simulink model "hip_controller_2026_03_03"  (R2024b)
settings: Solver=FixedStepAuto  StartTime=0.0  StopTime=simDuration  FixedStep=0.01  RelTol=1e-3  EnableMultiTasking=on
InitFcn:
  | breakp=[-1, -0.8, -0.6, -0.4, -0.2, -0.1, 0, 0.1, 0.2, 0.4, 0.6, 0.8, 1];
  | splinenew =[-1, -0.8, -0.6, -0.4, -0.2, -0.1, 0, 0, 0.005, 0.01, 0.015,0.02,0.025];
undefined symbols (not defined in the file or in its folder): Discrete, K, qbreak, Time
libraries: simulink x121, arduinolib x41, dspswit3 x21, ctrlSharedLib x2, dspfdesign x2, slpidlib x2
(part 4 of 7)

== system hip_controller_2026_03_03/Subsystem6/Right Motor Velocity/Subsystem ==
  Motor command : Inport
  SWITCH : Inport  Port=2
  CAN Pack1 : Subsystem
  CAN Transmit1 : arduinolib/CAN Transmit  Priority=1  inputDataType=Raw data  BlockingMode_=on  BlockTimeout_=1  outputStatus=off  identifierType=Standard (11-bit identifier)  messageId=3  msgLength=8  remoteFrame=off
      settings: SourceProductName=Common
  Constant7 : Constant  Value=0  OutDataTypeStr=single  SampleTime=0.01
  DISABLE1 : Constant  Value=269.7/18  OutDataTypeStr=single
  Data Type Conversion3 : DataTypeConversion  OutDataTypeStr=single  SaturateOnIntegerOverflow=off  RndMeth=Floor
  Demux1 : Demux  Outputs=5
  ENABLE1 : Constant  Value=14.975  OutDataTypeStr=single
  IsNaN : RelationalOperator  Operator=isNaN  OutDataTypeStr=boolean  RndMeth=Simplest  InputSameDT=off
  N-Sample Switch4 : dspswit3/N-Sample Switch  N=15  reset=on  TriggerType=Either edge  Ts=0.01
  Rate Transition : RateTransition  OutPortSampleTime=0.01
  Subsystem2 : Subsystem
  Switch : Switch  Criteria=u2 > Threshold  SaturateOnIntegerOverflow=off  InputSameDT=off
  Switch3 : Switch  Criteria=u2 > Threshold  SaturateOnIntegerOverflow=off  InputSameDT=off
  wires:
  Demux1/4 -> CAN Pack1/4(Kd)
  Data Type Conversion3/1 -> Subsystem2/2(Velocity)
  Switch3/1 -> Subsystem2/1(Enable)
  Demux1/1 -> CAN Pack1/1(Position)
  Motor command/1 -> Data Type Conversion3/1, IsNaN/1
  Demux1/5 -> CAN Pack1/5(Torque)
  ENABLE1/1 -> Switch3/1
  Demux1/2 -> CAN Pack1/2(Velocity)
  Rate Transition/1 -> N-Sample Switch4/3
  IsNaN/1 -> Switch/2
  DISABLE1/1 -> Switch3/3
  Subsystem2/1(Enter_motor_mode) -> N-Sample Switch4/1
  Demux1/3 -> CAN Pack1/3(Kp)
  N-Sample Switch4/1 -> Demux1/1
  Switch/1 -> Rate Transition/1, Switch3/2
  CAN Pack1/1(CAN Data) -> CAN Transmit1/1
  Subsystem2/2(Velocity_value) -> N-Sample Switch4/2
  Constant7/1 -> Switch/1
  SWITCH/1 -> Switch/3

== system hip_controller_2026_03_03/Initialize Function/Config_L /X=Z, Y=Y, Z=X/Enabled Subsystem ==
  Enable : EnablePort
  Compare To Constant1 : simulink/Logic and Bit Operations/Compare To Constant  relop===  const=0  OutDataTypeStr=boolean
  Constant2 : Constant  Value=0x06
  I2C Write6 : arduinolib/I2C Write  I2CModule=0  Mode=Master  SlaveAddress=0x28  SlaveByteOrder=BigEndian  Direction=Transmitter  RegisterAddressMode=on  RegisterAddress=0x41  SlaveDataType=uint8  DataLength=1  NoAck=off  RepeatedStart=off  OutputStatus=on  blockPlatform=ARDUINO
      settings: SourceProductName=Common
  Status : Outport
  wires:
  Constant2/1 -> I2C Write6/1
  I2C Write6/1 -> Compare To Constant1/1  "0: success"
  Compare To Constant1/1 -> Status/1

== system hip_controller_2026_03_03/Initialize Function/Config_L /Z = -Z/Write ==
  Enable : EnablePort
  Compare To Constant1 : simulink/Logic and Bit Operations/Compare To Constant  relop===  const=0  OutDataTypeStr=boolean
  Constant2 : Constant  Value=0x01
  I2C Write7 : arduinolib/I2C Write  I2CModule=0  Mode=Master  SlaveAddress=0x28  SlaveByteOrder=BigEndian  Direction=Transmitter  RegisterAddressMode=on  RegisterAddress=0x42  SlaveDataType=uint8  DataLength=1  NoAck=off  RepeatedStart=off  OutputStatus=on  blockPlatform=ARDUINO
      settings: SourceProductName=Common
  Status : Outport
  wires:
  Constant2/1 -> I2C Write7/1
  I2C Write7/1 -> Compare To Constant1/1  "0: success"
  Compare To Constant1/1 -> Status/1

== system hip_controller_2026_03_03/Initialize Function/Config_R/X=Z, Y=Y, Z=X/Enabled Subsystem ==
  Enable : EnablePort
  Compare To Constant1 : simulink/Logic and Bit Operations/Compare To Constant  relop===  const=0  OutDataTypeStr=boolean
  Constant2 : Constant  Value=0x06
  I2C Write6 : arduinolib/I2C Write  I2CModule=0  Mode=Master  SlaveAddress=0x29  SlaveByteOrder=BigEndian  Direction=Transmitter  RegisterAddressMode=on  RegisterAddress=0x41  SlaveDataType=uint8  DataLength=1  NoAck=off  RepeatedStart=off  OutputStatus=on  blockPlatform=ARDUINO
      settings: SourceProductName=Common
  Status : Outport
  wires:
  Constant2/1 -> I2C Write6/1
  I2C Write6/1 -> Compare To Constant1/1  "0: success"
  Compare To Constant1/1 -> Status/1

== system hip_controller_2026_03_03/Initialize Function/Config_R/Z = -Z/Write ==
  Enable : EnablePort
  Compare To Constant1 : simulink/Logic and Bit Operations/Compare To Constant  relop===  const=0  OutDataTypeStr=boolean
  Constant2 : Constant  Value=0x01
  I2C Write7 : arduinolib/I2C Write  I2CModule=0  Mode=Master  SlaveAddress=0x29  SlaveByteOrder=BigEndian  Direction=Transmitter  RegisterAddressMode=on  RegisterAddress=0x42  SlaveDataType=uint8  DataLength=1  NoAck=off  RepeatedStart=off  OutputStatus=on  blockPlatform=ARDUINO
      settings: SourceProductName=Common
  Status : Outport
  wires:
  Constant2/1 -> I2C Write7/1
  I2C Write7/1 -> Compare To Constant1/1  "0: success"
  Compare To Constant1/1 -> Status/1

== system hip_controller_2026_03_03/LEFT LEG1/Pos and Vel normalized/Subsystem4/If Action Subsystem ==
  Clock : Inport
  angle : Inport  Port=2
  Action Port : ActionPort
  Compare To Constant1 : simulink/Logic and Bit Operations/Compare To Constant  relop=>=  const=0.3  OutDataTypeStr=boolean
  Enabled Subsystem : Subsystem  TreatAsAtomicUnit=on
  Memory : Memory  InheritSampleTime=on
  Subtract : Sum  Inputs=+-
  Zero-Order Hold : ZeroOrderHold  SampleTime=-1
  Angle_max : Outport
  wires:
  Subtract/1 -> Compare To Constant1/1  "diff"
  Compare To Constant1/1 -> Enabled Subsystem/Enable  "enable"
  Enabled Subsystem/1(angle_out) -> Angle_max/1  "angle_out"
  angle/1 -> Enabled Subsystem/1(angle_in)
  Clock/1 -> Zero-Order Hold/1  "clock"
  Zero-Order Hold/1 -> Subtract/1, Memory/1  "clock_ZOH"
  Memory/1 -> Subtract/2  "clock_memory"

== system hip_controller_2026_03_03/LEFT LEG1/Pos and Vel normalized/Subsystem5/If Action Subsystem ==
  Angle : Inport
  Clock : Inport  Port=2
  Action Port : ActionPort
  Compare To Constant1 : simulink/Logic and Bit Operations/Compare To Constant  relop=>=  const=0.3  OutDataTypeStr=boolean
  Enabled Subsystem : Subsystem  TreatAsAtomicUnit=on
  Memory : Memory  InheritSampleTime=on
  Subtract : Sum  Inputs=+-
  Zero-Order Hold : ZeroOrderHold  SampleTime=-1
  Angle_min : Outport
  wires:
  Memory/1 -> Subtract/2  "clock_memory"
  Zero-Order Hold/1 -> Subtract/1, Memory/1  "clock_ZOH"
  Enabled Subsystem/1(angle_out) -> Angle_min/1  "angle_out"
  Compare To Constant1/1 -> Enabled Subsystem/Enable  "enable"
  Clock/1 -> Zero-Order Hold/1  "clock"
  Subtract/1 -> Compare To Constant1/1  "diff"
  Angle/1 -> Enabled Subsystem/1(angle_in)

== system hip_controller_2026_03_03/LEFT LEG1/Pos and Vel normalized/Subsystem6/If Action Subsystem ==
  Velocity : Inport
  Clock : Inport  Port=2
  Action Port : ActionPort
  Compare To Constant1 : simulink/Logic and Bit Operations/Compare To Constant  relop=>=  const=0.3  OutDataTypeStr=boolean
  Enabled Subsystem : Subsystem  TreatAsAtomicUnit=on
  Memory : Memory  InheritSampleTime=on
  Subtract : Sum  Inputs=+-
  Zero-Order Hold : ZeroOrderHold  SampleTime=-1
  Vel_min : Outport
  wires:
  Enabled Subsystem/1(vel_out) -> Vel_min/1  "angle_out"
  Memory/1 -> Subtract/2  "clock_memory"
  Velocity/1 -> Enabled Subsystem/1(vel_in)
  Zero-Order Hold/1 -> Subtract/1, Memory/1  "clock_ZOH"
  Clock/1 -> Zero-Order Hold/1  "clock"
  Subtract/1 -> Compare To Constant1/1  "diff"
  Compare To Constant1/1 -> Enabled Subsystem/Enable  "enable"

== system hip_controller_2026_03_03/LEFT LEG1/Pos and Vel normalized/Subsystem7/If Action Subsystem ==
  Velocity : Inport
  Clock : Inport  Port=2
  Action Port : ActionPort
  Compare To Constant1 : simulink/Logic and Bit Operations/Compare To Constant  relop=>=  const=0.3  OutDataTypeStr=boolean
  Enabled Subsystem : Subsystem  TreatAsAtomicUnit=on
  Memory : Memory  InheritSampleTime=on
  Subtract : Sum  Inputs=+-
  Zero-Order Hold : ZeroOrderHold  SampleTime=-1
  Vel_max : Outport
  wires:
  Memory/1 -> Subtract/2  "clock_memory"
  Compare To Constant1/1 -> Enabled Subsystem/Enable  "enable"
  Clock/1 -> Zero-Order Hold/1  "clock"
  Zero-Order Hold/1 -> Subtract/1, Memory/1  "clock_ZOH"
  Enabled Subsystem/1(vel_out) -> Vel_max/1  "angle_out"
  Subtract/1 -> Compare To Constant1/1  "diff"
  Velocity/1 -> Enabled Subsystem/1(vel_in)

== system hip_controller_2026_03_03/RIGHT_LEG1/Pos and Vel normalized/Subsystem4/If Action Subsystem ==
  Clock : Inport
  angle : Inport  Port=2
  Action Port : ActionPort
  Compare To Constant1 : simulink/Logic and Bit Operations/Compare To Constant  relop=>=  const=0.3  OutDataTypeStr=boolean
  Enabled Subsystem : Subsystem  TreatAsAtomicUnit=on
  Memory : Memory  InheritSampleTime=on
  Subtract : Sum  Inputs=+-
  Zero-Order Hold : ZeroOrderHold  SampleTime=-1
  Angle_max : Outport
  wires:
  Subtract/1 -> Compare To Constant1/1  "diff"
  Compare To Constant1/1 -> Enabled Subsystem/Enable  "enable"
  Enabled Subsystem/1(angle_out) -> Angle_max/1  "angle_out"
  angle/1 -> Enabled Subsystem/1(angle_in)
  Clock/1 -> Zero-Order Hold/1  "clock"
  Zero-Order Hold/1 -> Subtract/1, Memory/1  "clock_ZOH"
  Memory/1 -> Subtract/2  "clock_memory"

== system hip_controller_2026_03_03/RIGHT_LEG1/Pos and Vel normalized/Subsystem5/If Action Subsystem ==
  Angle : Inport
  Clock : Inport  Port=2
  Action Port : ActionPort
  Compare To Constant1 : simulink/Logic and Bit Operations/Compare To Constant  relop=>=  const=0.3  OutDataTypeStr=boolean
  Enabled Subsystem : Subsystem  TreatAsAtomicUnit=on
  Memory : Memory  InheritSampleTime=on
  Subtract : Sum  Inputs=+-
  Zero-Order Hold : ZeroOrderHold  SampleTime=-1
  Angle_min : Outport
  wires:
  Memory/1 -> Subtract/2  "clock_memory"
  Zero-Order Hold/1 -> Subtract/1, Memory/1  "clock_ZOH"
  Enabled Subsystem/1(angle_out) -> Angle_min/1  "angle_out"
  Compare To Constant1/1 -> Enabled Subsystem/Enable  "enable"
  Clock/1 -> Zero-Order Hold/1  "clock"
  Subtract/1 -> Compare To Constant1/1  "diff"
  Angle/1 -> Enabled Subsystem/1(angle_in)

== system hip_controller_2026_03_03/RIGHT_LEG1/Pos and Vel normalized/Subsystem6/If Action Subsystem ==
  Velocity : Inport
  Clock : Inport  Port=2
  Action Port : ActionPort
  Compare To Constant1 : simulink/Logic and Bit Operations/Compare To Constant  relop=>=  const=0.3  OutDataTypeStr=boolean
  Enabled Subsystem : Subsystem  TreatAsAtomicUnit=on
  Memory : Memory  InheritSampleTime=on
  Subtract : Sum  Inputs=+-
  Zero-Order Hold : ZeroOrderHold  SampleTime=-1
  Vel_min : Outport
  wires:
  Enabled Subsystem/1(vel_out) -> Vel_min/1  "angle_out"
  Memory/1 -> Subtract/2  "clock_memory"
  Velocity/1 -> Enabled Subsystem/1(vel_in)
  Zero-Order Hold/1 -> Subtract/1, Memory/1  "clock_ZOH"
  Clock/1 -> Zero-Order Hold/1  "clock"
  Subtract/1 -> Compare To Constant1/1  "diff"
  Compare To Constant1/1 -> Enabled Subsystem/Enable  "enable"

== system hip_controller_2026_03_03/RIGHT_LEG1/Pos and Vel normalized/Subsystem7/If Action Subsystem ==
  Velocity : Inport
  Clock : Inport  Port=2
  Action Port : ActionPort
  Compare To Constant1 : simulink/Logic and Bit Operations/Compare To Constant  relop=>=  const=0.3  OutDataTypeStr=boolean
  Enabled Subsystem : Subsystem  TreatAsAtomicUnit=on
  Memory : Memory  InheritSampleTime=on
  Subtract : Sum  Inputs=+-
  Zero-Order Hold : ZeroOrderHold  SampleTime=-1
  Vel_max : Outport
  wires:
  Memory/1 -> Subtract/2  "clock_memory"
  Compare To Constant1/1 -> Enabled Subsystem/Enable  "enable"
  Clock/1 -> Zero-Order Hold/1  "clock"
  Zero-Order Hold/1 -> Subtract/1, Memory/1  "clock_ZOH"
  Enabled Subsystem/1(vel_out) -> Vel_max/1  "angle_out"
  Subtract/1 -> Compare To Constant1/1  "diff"
  Velocity/1 -> Enabled Subsystem/1(vel_in)

== system hip_controller_2026_03_03/Subsystem3/Left Motor Velocity/Motor Actual Position Receive/CHINESE CORRECTION ==
  position : Inport
  Enable : EnablePort  StatesWhenEnabling=reset
  Abs : Abs  SaturateOnIntegerOverflow=off
  Constant2 : Constant
  Constant3 : Constant  Value=0
  Memory : Memory
  Subsystem : Subsystem
  Sum : Sum  Inputs=|+-
  Sum1 : Sum  Inputs=+-
  Switch1 : Switch  Criteria=u2 > Threshold  Threshold=20  SaturateOnIntegerOverflow=off  InputSameDT=off
  Out1 : Outport
  wires:
  Constant2/1 -> Switch1/1
  position/1 -> Sum1/1, Sum/1, Memory/1
  Sum/1 -> Abs/1, Subsystem/1(In1)
  Sum1/1 -> Out1/1
  Abs/1 -> Switch1/2
  Constant3/1 -> Switch1/3
  Switch1/1 -> Subsystem/Enable
  Memory/1 -> Sum/2
  Subsystem/1(Out1) -> Sum1/2

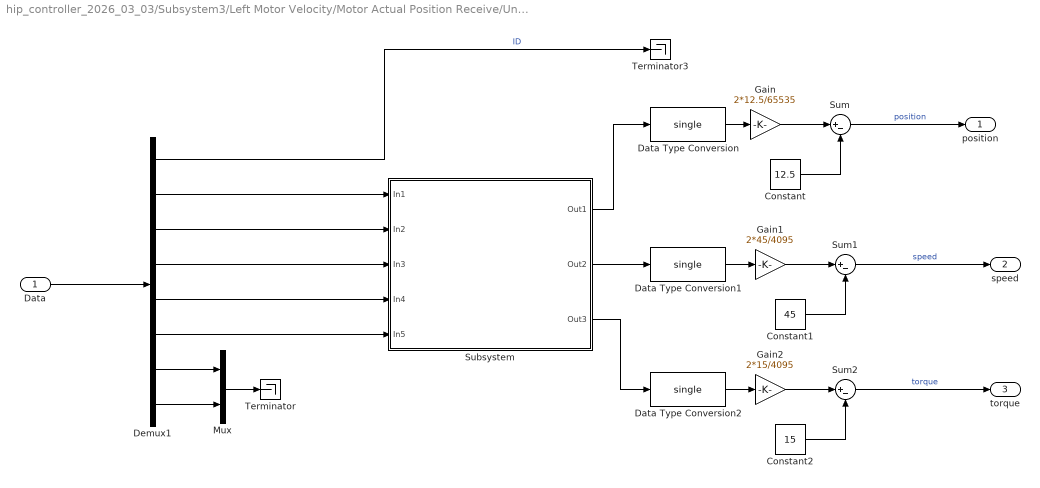
== system hip_controller_2026_03_03/Subsystem3/Left Motor Velocity/Motor Actual Position Receive/Unpack2 ==
  Data : Inport
  Constant : Constant  Value=12.5
  Constant1 : Constant  Value=45
  Constant2 : Constant  Value=15
  Data Type Conversion : DataTypeConversion  OutDataTypeStr=single  SaturateOnIntegerOverflow=off  RndMeth=Floor
  Data Type Conversion1 : DataTypeConversion  OutDataTypeStr=single  SaturateOnIntegerOverflow=off  RndMeth=Floor
  Data Type Conversion2 : DataTypeConversion  OutDataTypeStr=single  SaturateOnIntegerOverflow=off  RndMeth=Floor
  Demux1 : Demux  Outputs=8
  Gain : Gain  Gain=2*12.5/65535  RndMeth=Round
  Gain1 : Gain  Gain=2*45/4095  RndMeth=Round
  Gain2 : Gain  Gain=2*15/4095  RndMeth=Round
  Mux : Mux  Inputs=2
  Subsystem : Subsystem
  Sum : Sum  Inputs=|+-
  Sum1 : Sum  Inputs=|+-
  Sum2 : Sum  Inputs=|+-
  Terminator : Terminator
  Terminator3 : Terminator
  position : Outport
  speed : Outport  Port=2
  torque : Outport  Port=3
  wires:
  Demux1/1 -> Terminator3/1  "ID"
  Demux1/7 -> Mux/1
  Demux1/8 -> Mux/2
  Demux1/2 -> Subsystem/1(In1)
  Demux1/3 -> Subsystem/2(In2)
  Demux1/4 -> Subsystem/3(In3)
  Demux1/5 -> Subsystem/4(In4)
  Demux1/6 -> Subsystem/5(In5)
  Subsystem/1(Out1) -> Data Type Conversion/1
  Gain/1 -> Sum/1
  Constant/1 -> Sum/2
  Data Type Conversion/1 -> Gain/1
  Gain1/1 -> Sum1/1
  Data Type Conversion1/1 -> Gain1/1
  Constant1/1 -> Sum1/2
  Gain2/1 -> Sum2/1
  Data Type Conversion2/1 -> Gain2/1
  Constant2/1 -> Sum2/2
  Subsystem/2(Out2) -> Data Type Conversion1/1
  Subsystem/3(Out3) -> Data Type Conversion2/1
  Sum2/1 -> torque/1  "torque"
  Mux/1 -> Terminator/1
  Data/1 -> Demux1/1
  Sum/1 -> position/1  "position"
  Sum1/1 -> speed/1  "speed"

== system hip_controller_2026_03_03/Subsystem3/Left Motor Velocity/Subsystem/CAN Pack1 ==
  Position : Inport
  Velocity : Inport  Port=2
  Kp : Inport  Port=3
  Kd : Inport  Port=4
  Torque : Inport  Port=5
  Constant3 : Constant  Value=-12.5  OutDataTypeStr=single
  Constant4 : Constant  Value=-45  OutDataTypeStr=single
  Constant5 : Constant  Value=-15  OutDataTypeStr=single
  Gain : Gain  Gain=65535/(2*12.5)  OutDataTypeStr=uint16  RndMeth=Round
  Gain3 : Gain  Gain=4095/(2*45)  OutDataTypeStr=fixdt(0,12,0)  RndMeth=Round
  Gain4 : Gain  Gain=4095/500  OutDataTypeStr=fixdt(0,12,0)  RndMeth=Round
  Gain5 : Gain  Gain=4095/5  OutDataTypeStr=fixdt(0,12,0)  RndMeth=Round
  Gain6 : Gain  Gain=4095/(2*15)  OutDataTypeStr=fixdt(0,12,0)  RndMeth=Round
  Subsystem : Subsystem
  Sum3 : Sum  Inputs=|+-
  Sum4 : Sum  Inputs=|+-
  Sum5 : Sum  Inputs=|+-
  Vector Concatenate : Concatenate  NumInputs=8
  CAN Data : Outport
  wires:
  Velocity/1 -> Sum4/1
  Kp/1 -> Gain4/1
  Kd/1 -> Gain5/1
  Vector Concatenate/1 -> CAN Data/1
  Constant3/1 -> Sum3/2
  Sum3/1 -> Gain/1  "position"
  Position/1 -> Sum3/1
  Constant4/1 -> Sum4/2
  Constant5/1 -> Sum5/2
  Sum5/1 -> Gain6/1  "torque"
  Torque/1 -> Sum5/1
  Sum4/1 -> Gain3/1  "speed"
  Gain/1 -> Subsystem/1(p_int)
  Gain3/1 -> Subsystem/2(v_int)
  Gain4/1 -> Subsystem/3(kp_int)
  Gain5/1 -> Subsystem/4(kd_int)
  Gain6/1 -> Subsystem/5(t_int)
  Subsystem/1(Out2) -> Vector Concatenate/1
  Subsystem/2(Out1) -> Vector Concatenate/2
  Subsystem/4(Out4) -> Vector Concatenate/4
  Subsystem/5(Out5) -> Vector Concatenate/5
  Subsystem/6(Out6) -> Vector Concatenate/6
  Subsystem/7(Out7) -> Vector Concatenate/7
  Subsystem/3(Out3) -> Vector Concatenate/3
  Subsystem/8(Out8) -> Vector Concatenate/8

== system hip_controller_2026_03_03/Subsystem3/Left Motor Velocity/Subsystem/Subsystem2 ==
  Enable : Inport
  Velocity : Inport  Port=2
  Mux1 : Mux  Inputs=5
  Subsystem : Subsystem
  Subsystem2 : Subsystem
  Enter_motor_mode : Outport
  Velocity_value : Outport  Port=2
  wires:
  Subsystem2/3(Out3) -> Mux1/3
  Subsystem2/2(Out2) -> Mux1/2
  Subsystem2/4(Out4) -> Mux1/4
  Subsystem2/1(Out1) -> Mux1/1
  Subsystem/1(Out1) -> Velocity_value/1
  Mux1/1 -> Enter_motor_mode/1
  Enable/1 -> Mux1/5
  Velocity/1 -> Subsystem/1(In1)

== system hip_controller_2026_03_03/Subsystem3/Right Motor Velocity/Motor Actual Position Receive/CHINESE CORRECTION ==
  position : Inport
  Enable : EnablePort  StatesWhenEnabling=reset
  Abs : Abs  SaturateOnIntegerOverflow=off
  Constant2 : Constant
  Constant3 : Constant  Value=0
  Memory : Memory
  Subsystem : Subsystem
  Sum : Sum  Inputs=|+-
  Sum1 : Sum  Inputs=+-
  Switch1 : Switch  Criteria=u2 > Threshold  Threshold=20  SaturateOnIntegerOverflow=off  InputSameDT=off
  Out1 : Outport
  wires:
  Constant2/1 -> Switch1/1
  position/1 -> Sum1/1, Sum/1, Memory/1
  Sum/1 -> Abs/1, Subsystem/1(In1)
  Sum1/1 -> Out1/1
  Abs/1 -> Switch1/2
  Constant3/1 -> Switch1/3
  Switch1/1 -> Subsystem/Enable
  Memory/1 -> Sum/2
  Subsystem/1(Out1) -> Sum1/2

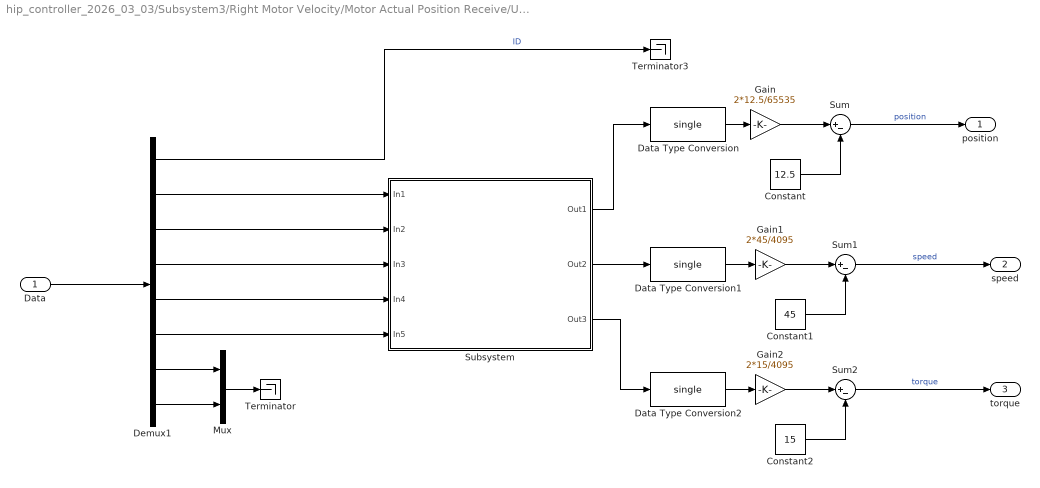
== system hip_controller_2026_03_03/Subsystem3/Right Motor Velocity/Motor Actual Position Receive/Unpack2 ==
  Data : Inport
  Constant : Constant  Value=12.5
  Constant1 : Constant  Value=45
  Constant2 : Constant  Value=15
  Data Type Conversion : DataTypeConversion  OutDataTypeStr=single  SaturateOnIntegerOverflow=off  RndMeth=Floor
  Data Type Conversion1 : DataTypeConversion  OutDataTypeStr=single  SaturateOnIntegerOverflow=off  RndMeth=Floor
  Data Type Conversion2 : DataTypeConversion  OutDataTypeStr=single  SaturateOnIntegerOverflow=off  RndMeth=Floor
  Demux1 : Demux  Outputs=8
  Gain : Gain  Gain=2*12.5/65535  RndMeth=Round
  Gain1 : Gain  Gain=2*45/4095  RndMeth=Round
  Gain2 : Gain  Gain=2*15/4095  RndMeth=Round
  Mux : Mux  Inputs=2
  Subsystem : Subsystem
  Sum : Sum  Inputs=|+-
  Sum1 : Sum  Inputs=|+-
  Sum2 : Sum  Inputs=|+-
  Terminator : Terminator
  Terminator3 : Terminator
  position : Outport
  speed : Outport  Port=2
  torque : Outport  Port=3
  wires:
  Demux1/1 -> Terminator3/1  "ID"
  Demux1/7 -> Mux/1
  Demux1/8 -> Mux/2
  Demux1/2 -> Subsystem/1(In1)
  Demux1/3 -> Subsystem/2(In2)
  Demux1/4 -> Subsystem/3(In3)
  Demux1/5 -> Subsystem/4(In4)
  Demux1/6 -> Subsystem/5(In5)
  Subsystem/1(Out1) -> Data Type Conversion/1
  Gain/1 -> Sum/1
  Constant/1 -> Sum/2
  Data Type Conversion/1 -> Gain/1
  Gain1/1 -> Sum1/1
  Data Type Conversion1/1 -> Gain1/1
  Constant1/1 -> Sum1/2
  Gain2/1 -> Sum2/1
  Data Type Conversion2/1 -> Gain2/1
  Constant2/1 -> Sum2/2
  Subsystem/2(Out2) -> Data Type Conversion1/1
  Subsystem/3(Out3) -> Data Type Conversion2/1
  Sum2/1 -> torque/1  "torque"
  Mux/1 -> Terminator/1
  Data/1 -> Demux1/1
  Sum/1 -> position/1  "position"
  Sum1/1 -> speed/1  "speed"

== system hip_controller_2026_03_03/Subsystem3/Right Motor Velocity/Subsystem/CAN Pack1 ==
  Position : Inport
  Velocity : Inport  Port=2
  Kp : Inport  Port=3
  Kd : Inport  Port=4
  Torque : Inport  Port=5
  Constant3 : Constant  Value=-12.5  OutDataTypeStr=single
  Constant4 : Constant  Value=-45  OutDataTypeStr=single
  Constant5 : Constant  Value=-15  OutDataTypeStr=single
  Gain : Gain  Gain=65535/(2*12.5)  OutDataTypeStr=uint16  RndMeth=Round
  Gain3 : Gain  Gain=4095/(2*45)  OutDataTypeStr=fixdt(0,12,0)  RndMeth=Round
  Gain4 : Gain  Gain=4095/500  OutDataTypeStr=fixdt(0,12,0)  RndMeth=Round
  Gain5 : Gain  Gain=4095/5  OutDataTypeStr=fixdt(0,12,0)  RndMeth=Round
  Gain6 : Gain  Gain=4095/(2*15)  OutDataTypeStr=fixdt(0,12,0)  RndMeth=Round
  Subsystem : Subsystem
  Sum3 : Sum  Inputs=|+-
  Sum4 : Sum  Inputs=|+-
  Sum5 : Sum  Inputs=|+-
  Vector Concatenate : Concatenate  NumInputs=8
  CAN Data : Outport
  wires:
  Velocity/1 -> Sum4/1
  Kp/1 -> Gain4/1
  Kd/1 -> Gain5/1
  Vector Concatenate/1 -> CAN Data/1
  Constant3/1 -> Sum3/2
  Sum3/1 -> Gain/1  "position"
  Position/1 -> Sum3/1
  Constant4/1 -> Sum4/2
  Constant5/1 -> Sum5/2
  Sum5/1 -> Gain6/1  "torque"
  Torque/1 -> Sum5/1
  Sum4/1 -> Gain3/1  "speed"
  Gain/1 -> Subsystem/1(p_int)
  Gain3/1 -> Subsystem/2(v_int)
  Gain4/1 -> Subsystem/3(kp_int)
  Gain5/1 -> Subsystem/4(kd_int)
  Gain6/1 -> Subsystem/5(t_int)
  Subsystem/1(Out2) -> Vector Concatenate/1
  Subsystem/2(Out1) -> Vector Concatenate/2
  Subsystem/4(Out4) -> Vector Concatenate/4
  Subsystem/5(Out5) -> Vector Concatenate/5
  Subsystem/6(Out6) -> Vector Concatenate/6
  Subsystem/7(Out7) -> Vector Concatenate/7
  Subsystem/3(Out3) -> Vector Concatenate/3
  Subsystem/8(Out8) -> Vector Concatenate/8

== system hip_controller_2026_03_03/Subsystem3/Right Motor Velocity/Subsystem/Subsystem2 ==
  Enable : Inport
  Velocity : Inport  Port=2
  Mux1 : Mux  Inputs=5
  Subsystem : Subsystem
  Subsystem2 : Subsystem
  Enter_motor_mode : Outport
  Velocity_value : Outport  Port=2
  wires:
  Subsystem2/3(Out3) -> Mux1/3
  Subsystem2/2(Out2) -> Mux1/2
  Subsystem2/4(Out4) -> Mux1/4
  Subsystem2/1(Out1) -> Mux1/1
  Subsystem/1(Out1) -> Velocity_value/1
  Mux1/1 -> Enter_motor_mode/1
  Enable/1 -> Mux1/5
  Velocity/1 -> Subsystem/1(In1)

== system hip_controller_2026_03_03/Subsystem4/Left Motor Velocity/Motor Actual Position Receive/CHINESE CORRECTION ==
  position : Inport
  Enable : EnablePort  StatesWhenEnabling=reset
  Abs : Abs  SaturateOnIntegerOverflow=off
  Constant2 : Constant
  Constant3 : Constant  Value=0
  Memory : Memory
  Subsystem : Subsystem
  Sum : Sum  Inputs=|+-
  Sum1 : Sum  Inputs=+-
  Switch1 : Switch  Criteria=u2 > Threshold  Threshold=20  SaturateOnIntegerOverflow=off  InputSameDT=off
  Out1 : Outport
  wires:
  Constant2/1 -> Switch1/1
  position/1 -> Sum1/1, Sum/1, Memory/1
  Sum/1 -> Abs/1, Subsystem/1(In1)
  Sum1/1 -> Out1/1
  Abs/1 -> Switch1/2
  Constant3/1 -> Switch1/3
  Switch1/1 -> Subsystem/Enable
  Memory/1 -> Sum/2
  Subsystem/1(Out1) -> Sum1/2

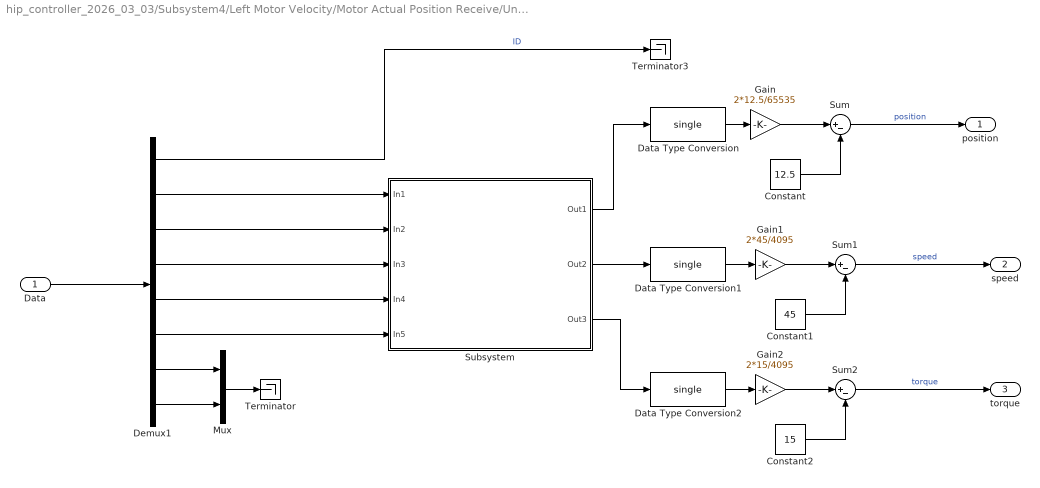
== system hip_controller_2026_03_03/Subsystem4/Left Motor Velocity/Motor Actual Position Receive/Unpack2 ==
  Data : Inport
  Constant : Constant  Value=12.5
  Constant1 : Constant  Value=45
  Constant2 : Constant  Value=15
  Data Type Conversion : DataTypeConversion  OutDataTypeStr=single  SaturateOnIntegerOverflow=off  RndMeth=Floor
  Data Type Conversion1 : DataTypeConversion  OutDataTypeStr=single  SaturateOnIntegerOverflow=off  RndMeth=Floor
  Data Type Conversion2 : DataTypeConversion  OutDataTypeStr=single  SaturateOnIntegerOverflow=off  RndMeth=Floor
  Demux1 : Demux  Outputs=8
  Gain : Gain  Gain=2*12.5/65535  RndMeth=Round
  Gain1 : Gain  Gain=2*45/4095  RndMeth=Round
  Gain2 : Gain  Gain=2*15/4095  RndMeth=Round
  Mux : Mux  Inputs=2
  Subsystem : Subsystem
  Sum : Sum  Inputs=|+-
  Sum1 : Sum  Inputs=|+-
  Sum2 : Sum  Inputs=|+-
  Terminator : Terminator
  Terminator3 : Terminator
  position : Outport
  speed : Outport  Port=2
  torque : Outport  Port=3
  wires:
  Demux1/1 -> Terminator3/1  "ID"
  Demux1/7 -> Mux/1
  Demux1/8 -> Mux/2
  Demux1/2 -> Subsystem/1(In1)
  Demux1/3 -> Subsystem/2(In2)
  Demux1/4 -> Subsystem/3(In3)
  Demux1/5 -> Subsystem/4(In4)
  Demux1/6 -> Subsystem/5(In5)
  Subsystem/1(Out1) -> Data Type Conversion/1
  Gain/1 -> Sum/1
  Constant/1 -> Sum/2
  Data Type Conversion/1 -> Gain/1
  Gain1/1 -> Sum1/1
  Data Type Conversion1/1 -> Gain1/1
  Constant1/1 -> Sum1/2
  Gain2/1 -> Sum2/1
  Data Type Conversion2/1 -> Gain2/1
  Constant2/1 -> Sum2/2
  Subsystem/2(Out2) -> Data Type Conversion1/1
  Subsystem/3(Out3) -> Data Type Conversion2/1
  Sum2/1 -> torque/1  "torque"
  Mux/1 -> Terminator/1
  Data/1 -> Demux1/1
  Sum/1 -> position/1  "position"
  Sum1/1 -> speed/1  "speed"

== system hip_controller_2026_03_03/Subsystem4/Left Motor Velocity/Subsystem/CAN Pack1 ==
  Position : Inport
  Velocity : Inport  Port=2
  Kp : Inport  Port=3
  Kd : Inport  Port=4
  Torque : Inport  Port=5
  Constant3 : Constant  Value=-12.5  OutDataTypeStr=single
  Constant4 : Constant  Value=-45  OutDataTypeStr=single
  Constant5 : Constant  Value=-15  OutDataTypeStr=single
  Gain : Gain  Gain=65535/(2*12.5)  OutDataTypeStr=uint16  RndMeth=Round
  Gain3 : Gain  Gain=4095/(2*45)  OutDataTypeStr=fixdt(0,12,0)  RndMeth=Round
  Gain4 : Gain  Gain=4095/500  OutDataTypeStr=fixdt(0,12,0)  RndMeth=Round
  Gain5 : Gain  Gain=4095/5  OutDataTypeStr=fixdt(0,12,0)  RndMeth=Round
  Gain6 : Gain  Gain=4095/(2*15)  OutDataTypeStr=fixdt(0,12,0)  RndMeth=Round
  Subsystem : Subsystem
  Sum3 : Sum  Inputs=|+-
  Sum4 : Sum  Inputs=|+-
  Sum5 : Sum  Inputs=|+-
  Vector Concatenate : Concatenate  NumInputs=8
  CAN Data : Outport
  wires:
  Velocity/1 -> Sum4/1
  Kp/1 -> Gain4/1
  Kd/1 -> Gain5/1
  Vector Concatenate/1 -> CAN Data/1
  Constant3/1 -> Sum3/2
  Sum3/1 -> Gain/1  "position"
  Position/1 -> Sum3/1
  Constant4/1 -> Sum4/2
  Constant5/1 -> Sum5/2
  Sum5/1 -> Gain6/1  "torque"
  Torque/1 -> Sum5/1
  Sum4/1 -> Gain3/1  "speed"
  Gain/1 -> Subsystem/1(p_int)
  Gain3/1 -> Subsystem/2(v_int)
  Gain4/1 -> Subsystem/3(kp_int)
  Gain5/1 -> Subsystem/4(kd_int)
  Gain6/1 -> Subsystem/5(t_int)
  Subsystem/1(Out2) -> Vector Concatenate/1
  Subsystem/2(Out1) -> Vector Concatenate/2
  Subsystem/4(Out4) -> Vector Concatenate/4
  Subsystem/5(Out5) -> Vector Concatenate/5
  Subsystem/6(Out6) -> Vector Concatenate/6
  Subsystem/7(Out7) -> Vector Concatenate/7
  Subsystem/3(Out3) -> Vector Concatenate/3
  Subsystem/8(Out8) -> Vector Concatenate/8

== system hip_controller_2026_03_03/Subsystem4/Left Motor Velocity/Subsystem/Subsystem2 ==
  Enable : Inport
  Velocity : Inport  Port=2
  Mux1 : Mux  Inputs=5
  Subsystem : Subsystem
  Subsystem2 : Subsystem
  Enter_motor_mode : Outport
  Velocity_value : Outport  Port=2
  wires:
  Subsystem2/3(Out3) -> Mux1/3
  Subsystem2/2(Out2) -> Mux1/2
  Subsystem2/4(Out4) -> Mux1/4
  Subsystem2/1(Out1) -> Mux1/1
  Subsystem/1(Out1) -> Velocity_value/1
  Mux1/1 -> Enter_motor_mode/1
  Enable/1 -> Mux1/5
  Velocity/1 -> Subsystem/1(In1)

== system hip_controller_2026_03_03/Subsystem4/Right Motor Velocity/Motor Actual Position Receive/CHINESE CORRECTION ==
  position : Inport
  Enable : EnablePort  StatesWhenEnabling=reset
  Abs : Abs  SaturateOnIntegerOverflow=off
  Constant2 : Constant
  Constant3 : Constant  Value=0
  Memory : Memory
  Subsystem : Subsystem
  Sum : Sum  Inputs=|+-
  Sum1 : Sum  Inputs=+-
  Switch1 : Switch  Criteria=u2 > Threshold  Threshold=20  SaturateOnIntegerOverflow=off  InputSameDT=off
  Out1 : Outport
  wires:
  Constant2/1 -> Switch1/1
  position/1 -> Sum1/1, Sum/1, Memory/1
  Sum/1 -> Abs/1, Subsystem/1(In1)
  Sum1/1 -> Out1/1
  Abs/1 -> Switch1/2
  Constant3/1 -> Switch1/3
  Switch1/1 -> Subsystem/Enable
  Memory/1 -> Sum/2
  Subsystem/1(Out1) -> Sum1/2

== system hip_controller_2026_03_03/Subsystem4/Right Motor Velocity/Motor Actual Position Receive/Unpack2 ==
  Data : Inport
  Constant : Constant  Value=12.5
  Constant1 : Constant  Value=45
  Constant2 : Constant  Value=15
  Data Type Conversion : DataTypeConversion  OutDataTypeStr=single  SaturateOnIntegerOverflow=off  RndMeth=Floor
  Data Type Conversion1 : DataTypeConversion  OutDataTypeStr=single  SaturateOnIntegerOverflow=off  RndMeth=Floor
  Data Type Conversion2 : DataTypeConversion  OutDataTypeStr=single  SaturateOnIntegerOverflow=off  RndMeth=Floor
  Demux1 : Demux  Outputs=8
  Gain : Gain  Gain=2*12.5/65535  RndMeth=Round
  Gain1 : Gain  Gain=2*45/4095  RndMeth=Round
  Gain2 : Gain  Gain=2*15/4095  RndMeth=Round
  Mux : Mux  Inputs=2
  Subsystem : Subsystem
  Sum : Sum  Inputs=|+-
  Sum1 : Sum  Inputs=|+-
  Sum2 : Sum  Inputs=|+-
  Terminator : Terminator
  Terminator3 : Terminator
  position : Outport
  speed : Outport  Port=2
  torque : Outport  Port=3
  wires:
  Demux1/1 -> Terminator3/1  "ID"
  Demux1/7 -> Mux/1
  Demux1/8 -> Mux/2
  Demux1/2 -> Subsystem/1(In1)
  Demux1/3 -> Subsystem/2(In2)
  Demux1/4 -> Subsystem/3(In3)
  Demux1/5 -> Subsystem/4(In4)
  Demux1/6 -> Subsystem/5(In5)
  Subsystem/1(Out1) -> Data Type Conversion/1
  Gain/1 -> Sum/1
  Constant/1 -> Sum/2
  Data Type Conversion/1 -> Gain/1
  Gain1/1 -> Sum1/1
  Data Type Conversion1/1 -> Gain1/1
  Constant1/1 -> Sum1/2
  Gain2/1 -> Sum2/1
  Data Type Conversion2/1 -> Gain2/1
  Constant2/1 -> Sum2/2
  Subsystem/2(Out2) -> Data Type Conversion1/1
  Subsystem/3(Out3) -> Data Type Conversion2/1
  Sum2/1 -> torque/1  "torque"
  Mux/1 -> Terminator/1
  Data/1 -> Demux1/1
  Sum/1 -> position/1  "position"
  Sum1/1 -> speed/1  "speed"

== system hip_controller_2026_03_03/Subsystem4/Right Motor Velocity/Subsystem/CAN Pack1 ==
  Position : Inport
  Velocity : Inport  Port=2
  Kp : Inport  Port=3
  Kd : Inport  Port=4
  Torque : Inport  Port=5
  Constant3 : Constant  Value=-12.5  OutDataTypeStr=single
  Constant4 : Constant  Value=-45  OutDataTypeStr=single
  Constant5 : Constant  Value=-15  OutDataTypeStr=single
  Gain : Gain  Gain=65535/(2*12.5)  OutDataTypeStr=uint16  RndMeth=Round
  Gain3 : Gain  Gain=4095/(2*45)  OutDataTypeStr=fixdt(0,12,0)  RndMeth=Round
  Gain4 : Gain  Gain=4095/500  OutDataTypeStr=fixdt(0,12,0)  RndMeth=Round
  Gain5 : Gain  Gain=4095/5  OutDataTypeStr=fixdt(0,12,0)  RndMeth=Round
  Gain6 : Gain  Gain=4095/(2*15)  OutDataTypeStr=fixdt(0,12,0)  RndMeth=Round
  Subsystem : Subsystem
  Sum3 : Sum  Inputs=|+-
  Sum4 : Sum  Inputs=|+-
  Sum5 : Sum  Inputs=|+-
  Vector Concatenate : Concatenate  NumInputs=8
  CAN Data : Outport
  wires:
  Velocity/1 -> Sum4/1
  Kp/1 -> Gain4/1
  Kd/1 -> Gain5/1
  Vector Concatenate/1 -> CAN Data/1
  Constant3/1 -> Sum3/2
  Sum3/1 -> Gain/1  "position"
  Position/1 -> Sum3/1
  Constant4/1 -> Sum4/2
  Constant5/1 -> Sum5/2
  Sum5/1 -> Gain6/1  "torque"
  Torque/1 -> Sum5/1
  Sum4/1 -> Gain3/1  "speed"
  Gain/1 -> Subsystem/1(p_int)
  Gain3/1 -> Subsystem/2(v_int)
  Gain4/1 -> Subsystem/3(kp_int)
  Gain5/1 -> Subsystem/4(kd_int)
  Gain6/1 -> Subsystem/5(t_int)
  Subsystem/1(Out2) -> Vector Concatenate/1
  Subsystem/2(Out1) -> Vector Concatenate/2
  Subsystem/4(Out4) -> Vector Concatenate/4
  Subsystem/5(Out5) -> Vector Concatenate/5
  Subsystem/6(Out6) -> Vector Concatenate/6
  Subsystem/7(Out7) -> Vector Concatenate/7
  Subsystem/3(Out3) -> Vector Concatenate/3
  Subsystem/8(Out8) -> Vector Concatenate/8

== system hip_controller_2026_03_03/Subsystem4/Right Motor Velocity/Subsystem/Subsystem2 ==
  Enable : Inport
  Velocity : Inport  Port=2
  Mux1 : Mux  Inputs=5
  Subsystem : Subsystem
  Subsystem2 : Subsystem
  Enter_motor_mode : Outport
  Velocity_value : Outport  Port=2
  wires:
  Subsystem2/3(Out3) -> Mux1/3
  Subsystem2/2(Out2) -> Mux1/2
  Subsystem2/4(Out4) -> Mux1/4
  Subsystem2/1(Out1) -> Mux1/1
  Subsystem/1(Out1) -> Velocity_value/1
  Mux1/1 -> Enter_motor_mode/1
  Enable/1 -> Mux1/5
  Velocity/1 -> Subsystem/1(In1)

== system hip_controller_2026_03_03/Subsystem5/Left Motor Velocity1/Motor Actual Position Receive/CHINESE CORRECTION ==
  position : Inport
  Enable : EnablePort  StatesWhenEnabling=reset
  Abs : Abs  SaturateOnIntegerOverflow=off
  Constant2 : Constant
  Constant3 : Constant  Value=0
  Memory : Memory
  Subsystem : Subsystem
  Sum : Sum  Inputs=|+-
  Sum1 : Sum  Inputs=+-
  Switch1 : Switch  Criteria=u2 > Threshold  Threshold=20  SaturateOnIntegerOverflow=off  InputSameDT=off
  Out1 : Outport
  wires:
  Constant2/1 -> Switch1/1
  position/1 -> Sum1/1, Sum/1, Memory/1
  Sum/1 -> Abs/1, Subsystem/1(In1)
  Sum1/1 -> Out1/1
  Abs/1 -> Switch1/2
  Constant3/1 -> Switch1/3
  Switch1/1 -> Subsystem/Enable
  Memory/1 -> Sum/2
  Subsystem/1(Out1) -> Sum1/2

== system hip_controller_2026_03_03/Subsystem5/Left Motor Velocity1/Motor Actual Position Receive/Unpack2 ==
  Data : Inport
  Constant : Constant  Value=12.5
  Constant1 : Constant  Value=45
  Constant2 : Constant  Value=15
  Data Type Conversion : DataTypeConversion  OutDataTypeStr=single  SaturateOnIntegerOverflow=off  RndMeth=Floor
  Data Type Conversion1 : DataTypeConversion  OutDataTypeStr=single  SaturateOnIntegerOverflow=off  RndMeth=Floor
  Data Type Conversion2 : DataTypeConversion  OutDataTypeStr=single  SaturateOnIntegerOverflow=off  RndMeth=Floor
  Demux1 : Demux  Outputs=8
  Gain : Gain  Gain=2*12.5/65535  RndMeth=Round
  Gain1 : Gain  Gain=2*45/4095  RndMeth=Round
  Gain2 : Gain  Gain=2*15/4095  RndMeth=Round
  Mux : Mux  Inputs=2
  Subsystem : Subsystem
  Sum : Sum  Inputs=|+-
  Sum1 : Sum  Inputs=|+-
  Sum2 : Sum  Inputs=|+-
  Terminator : Terminator
  Terminator3 : Terminator
  position : Outport
  speed : Outport  Port=2
  torque : Outport  Port=3
  wires:
  Demux1/1 -> Terminator3/1  "ID"
  Demux1/7 -> Mux/1
  Demux1/8 -> Mux/2
  Demux1/2 -> Subsystem/1(In1)
  Demux1/3 -> Subsystem/2(In2)
  Demux1/4 -> Subsystem/3(In3)
  Demux1/5 -> Subsystem/4(In4)
  Demux1/6 -> Subsystem/5(In5)
  Subsystem/1(Out1) -> Data Type Conversion/1
  Gain/1 -> Sum/1
  Constant/1 -> Sum/2
  Data Type Conversion/1 -> Gain/1
  Gain1/1 -> Sum1/1
  Data Type Conversion1/1 -> Gain1/1
  Constant1/1 -> Sum1/2
  Gain2/1 -> Sum2/1
  Data Type Conversion2/1 -> Gain2/1
  Constant2/1 -> Sum2/2
  Subsystem/2(Out2) -> Data Type Conversion1/1
  Subsystem/3(Out3) -> Data Type Conversion2/1
  Sum2/1 -> torque/1  "torque"
  Mux/1 -> Terminator/1
  Data/1 -> Demux1/1
  Sum/1 -> position/1  "position"
  Sum1/1 -> speed/1  "speed"

== system hip_controller_2026_03_03/Subsystem5/Left Motor Velocity1/Subsystem/CAN Pack1 ==
  Position : Inport
  Velocity : Inport  Port=2
  Kp : Inport  Port=3
  Kd : Inport  Port=4
  Torque : Inport  Port=5
  Constant3 : Constant  Value=-12.5  OutDataTypeStr=single
  Constant4 : Constant  Value=-45  OutDataTypeStr=single
  Constant5 : Constant  Value=-15  OutDataTypeStr=single
  Gain : Gain  Gain=65535/(2*12.5)  OutDataTypeStr=uint16  RndMeth=Round
  Gain3 : Gain  Gain=4095/(2*45)  OutDataTypeStr=fixdt(0,12,0)  RndMeth=Round
  Gain4 : Gain  Gain=4095/500  OutDataTypeStr=fixdt(0,12,0)  RndMeth=Round
  Gain5 : Gain  Gain=4095/5  OutDataTypeStr=fixdt(0,12,0)  RndMeth=Round
  Gain6 : Gain  Gain=4095/(2*15)  OutDataTypeStr=fixdt(0,12,0)  RndMeth=Round
  Subsystem : Subsystem
  Sum3 : Sum  Inputs=|+-
  Sum4 : Sum  Inputs=|+-
  Sum5 : Sum  Inputs=|+-
  Vector Concatenate : Concatenate  NumInputs=8
  CAN Data : Outport
  wires:
  Velocity/1 -> Sum4/1
  Kp/1 -> Gain4/1
  Kd/1 -> Gain5/1
  Vector Concatenate/1 -> CAN Data/1
  Constant3/1 -> Sum3/2
  Sum3/1 -> Gain/1  "position"
  Position/1 -> Sum3/1
  Constant4/1 -> Sum4/2
  Constant5/1 -> Sum5/2
  Sum5/1 -> Gain6/1  "torque"
  Torque/1 -> Sum5/1
  Sum4/1 -> Gain3/1  "speed"
  Gain/1 -> Subsystem/1(p_int)
  Gain3/1 -> Subsystem/2(v_int)
  Gain4/1 -> Subsystem/3(kp_int)
  Gain5/1 -> Subsystem/4(kd_int)
  Gain6/1 -> Subsystem/5(t_int)
  Subsystem/1(Out2) -> Vector Concatenate/1
  Subsystem/2(Out1) -> Vector Concatenate/2
  Subsystem/4(Out4) -> Vector Concatenate/4
  Subsystem/5(Out5) -> Vector Concatenate/5
  Subsystem/6(Out6) -> Vector Concatenate/6
  Subsystem/7(Out7) -> Vector Concatenate/7
  Subsystem/3(Out3) -> Vector Concatenate/3
  Subsystem/8(Out8) -> Vector Concatenate/8

== system hip_controller_2026_03_03/Subsystem5/Left Motor Velocity1/Subsystem/Subsystem2 ==
  Enable : Inport
  Velocity : Inport  Port=2
  Mux1 : Mux  Inputs=5
  Subsystem : Subsystem
  Subsystem2 : Subsystem
  Enter_motor_mode : Outport
  Velocity_value : Outport  Port=2
  wires:
  Subsystem2/3(Out3) -> Mux1/3
  Subsystem2/2(Out2) -> Mux1/2
  Subsystem2/4(Out4) -> Mux1/4
  Subsystem2/1(Out1) -> Mux1/1
  Subsystem/1(Out1) -> Velocity_value/1
  Mux1/1 -> Enter_motor_mode/1
  Enable/1 -> Mux1/5
  Velocity/1 -> Subsystem/1(In1)

== system hip_controller_2026_03_03/Subsystem5/Right Motor Velocity1/Motor Actual Position Receive/CHINESE CORRECTION ==
  position : Inport
  Enable : EnablePort  StatesWhenEnabling=reset
  Abs : Abs  SaturateOnIntegerOverflow=off
  Constant2 : Constant
  Constant3 : Constant  Value=0
  Memory : Memory
  Subsystem : Subsystem
  Sum : Sum  Inputs=|+-
  Sum1 : Sum  Inputs=+-
  Switch1 : Switch  Criteria=u2 > Threshold  Threshold=20  SaturateOnIntegerOverflow=off  InputSameDT=off
  Out1 : Outport
  wires:
  Constant2/1 -> Switch1/1
  position/1 -> Sum1/1, Sum/1, Memory/1
  Sum/1 -> Abs/1, Subsystem/1(In1)
  Sum1/1 -> Out1/1
  Abs/1 -> Switch1/2
  Constant3/1 -> Switch1/3
  Switch1/1 -> Subsystem/Enable
  Memory/1 -> Sum/2
  Subsystem/1(Out1) -> Sum1/2

== system hip_controller_2026_03_03/Subsystem5/Right Motor Velocity1/Motor Actual Position Receive/Unpack2 ==
  Data : Inport
  Constant : Constant  Value=12.5
  Constant1 : Constant  Value=45
  Constant2 : Constant  Value=15
  Data Type Conversion : DataTypeConversion  OutDataTypeStr=single  SaturateOnIntegerOverflow=off  RndMeth=Floor
  Data Type Conversion1 : DataTypeConversion  OutDataTypeStr=single  SaturateOnIntegerOverflow=off  RndMeth=Floor
  Data Type Conversion2 : DataTypeConversion  OutDataTypeStr=single  SaturateOnIntegerOverflow=off  RndMeth=Floor
  Demux1 : Demux  Outputs=8
  Gain : Gain  Gain=2*12.5/65535  RndMeth=Round
  Gain1 : Gain  Gain=2*45/4095  RndMeth=Round
  Gain2 : Gain  Gain=2*15/4095  RndMeth=Round
  Mux : Mux  Inputs=2
  Subsystem : Subsystem
  Sum : Sum  Inputs=|+-
  Sum1 : Sum  Inputs=|+-
  Sum2 : Sum  Inputs=|+-
  Terminator : Terminator
  Terminator3 : Terminator
  position : Outport
  speed : Outport  Port=2
  torque : Outport  Port=3
  wires:
  Demux1/1 -> Terminator3/1  "ID"
  Demux1/7 -> Mux/1
  Demux1/8 -> Mux/2
  Demux1/2 -> Subsystem/1(In1)
  Demux1/3 -> Subsystem/2(In2)
  Demux1/4 -> Subsystem/3(In3)
  Demux1/5 -> Subsystem/4(In4)
  Demux1/6 -> Subsystem/5(In5)
  Subsystem/1(Out1) -> Data Type Conversion/1
  Gain/1 -> Sum/1
  Constant/1 -> Sum/2
  Data Type Conversion/1 -> Gain/1
  Gain1/1 -> Sum1/1
  Data Type Conversion1/1 -> Gain1/1
  Constant1/1 -> Sum1/2
  Gain2/1 -> Sum2/1
  Data Type Conversion2/1 -> Gain2/1
  Constant2/1 -> Sum2/2
  Subsystem/2(Out2) -> Data Type Conversion1/1
  Subsystem/3(Out3) -> Data Type Conversion2/1
  Sum2/1 -> torque/1  "torque"
  Mux/1 -> Terminator/1
  Data/1 -> Demux1/1
  Sum/1 -> position/1  "position"
  Sum1/1 -> speed/1  "speed"

== system hip_controller_2026_03_03/Subsystem5/Right Motor Velocity1/Subsystem/CAN Pack1 ==
  Position : Inport
  Velocity : Inport  Port=2
  Kp : Inport  Port=3
  Kd : Inport  Port=4
  Torque : Inport  Port=5
  Constant3 : Constant  Value=-12.5  OutDataTypeStr=single
  Constant4 : Constant  Value=-45  OutDataTypeStr=single
  Constant5 : Constant  Value=-15  OutDataTypeStr=single
  Gain : Gain  Gain=65535/(2*12.5)  OutDataTypeStr=uint16  RndMeth=Round
  Gain3 : Gain  Gain=4095/(2*45)  OutDataTypeStr=fixdt(0,12,0)  RndMeth=Round
  Gain4 : Gain  Gain=4095/500  OutDataTypeStr=fixdt(0,12,0)  RndMeth=Round
  Gain5 : Gain  Gain=4095/5  OutDataTypeStr=fixdt(0,12,0)  RndMeth=Round
  Gain6 : Gain  Gain=4095/(2*15)  OutDataTypeStr=fixdt(0,12,0)  RndMeth=Round
  Subsystem : Subsystem
  Sum3 : Sum  Inputs=|+-
  Sum4 : Sum  Inputs=|+-
  Sum5 : Sum  Inputs=|+-
  Vector Concatenate : Concatenate  NumInputs=8
  CAN Data : Outport
  wires:
  Velocity/1 -> Sum4/1
  Kp/1 -> Gain4/1
  Kd/1 -> Gain5/1
  Vector Concatenate/1 -> CAN Data/1
  Constant3/1 -> Sum3/2
  Sum3/1 -> Gain/1  "position"
  Position/1 -> Sum3/1
  Constant4/1 -> Sum4/2
  Constant5/1 -> Sum5/2
  Sum5/1 -> Gain6/1  "torque"
  Torque/1 -> Sum5/1
  Sum4/1 -> Gain3/1  "speed"
  Gain/1 -> Subsystem/1(p_int)
  Gain3/1 -> Subsystem/2(v_int)
  Gain4/1 -> Subsystem/3(kp_int)
  Gain5/1 -> Subsystem/4(kd_int)
  Gain6/1 -> Subsystem/5(t_int)
  Subsystem/1(Out2) -> Vector Concatenate/1
  Subsystem/2(Out1) -> Vector Concatenate/2
  Subsystem/4(Out4) -> Vector Concatenate/4
  Subsystem/5(Out5) -> Vector Concatenate/5
  Subsystem/6(Out6) -> Vector Concatenate/6
  Subsystem/7(Out7) -> Vector Concatenate/7
  Subsystem/3(Out3) -> Vector Concatenate/3
  Subsystem/8(Out8) -> Vector Concatenate/8

== system hip_controller_2026_03_03/Subsystem5/Right Motor Velocity1/Subsystem/Subsystem2 ==
  Enable : Inport
  Velocity : Inport  Port=2
  Mux1 : Mux  Inputs=5
  Subsystem : Subsystem
  Subsystem2 : Subsystem
  Enter_motor_mode : Outport
  Velocity_value : Outport  Port=2
  wires:
  Subsystem2/3(Out3) -> Mux1/3
  Subsystem2/2(Out2) -> Mux1/2
  Subsystem2/4(Out4) -> Mux1/4
  Subsystem2/1(Out1) -> Mux1/1
  Subsystem/1(Out1) -> Velocity_value/1
  Mux1/1 -> Enter_motor_mode/1
  Enable/1 -> Mux1/5
  Velocity/1 -> Subsystem/1(In1)

== system hip_controller_2026_03_03/Subsystem6/Left Motor Velocity/Motor Actual Position Receive/CHINESE CORRECTION ==
  position : Inport
  Enable : EnablePort  StatesWhenEnabling=reset
  Abs : Abs  SaturateOnIntegerOverflow=off
  Constant2 : Constant
  Constant3 : Constant  Value=0
  Memory : Memory
  Subsystem : Subsystem
  Sum : Sum  Inputs=|+-
  Sum1 : Sum  Inputs=+-
  Switch1 : Switch  Criteria=u2 > Threshold  Threshold=20  SaturateOnIntegerOverflow=off  InputSameDT=off
  Out1 : Outport
  wires:
  Constant2/1 -> Switch1/1
  position/1 -> Sum1/1, Sum/1, Memory/1
  Sum/1 -> Abs/1, Subsystem/1(In1)
  Sum1/1 -> Out1/1
  Abs/1 -> Switch1/2
  Constant3/1 -> Switch1/3
  Switch1/1 -> Subsystem/Enable
  Memory/1 -> Sum/2
  Subsystem/1(Out1) -> Sum1/2

== system hip_controller_2026_03_03/Subsystem6/Left Motor Velocity/Motor Actual Position Receive/Unpack2 ==
  Data : Inport
  Constant : Constant  Value=12.5
  Constant1 : Constant  Value=45
  Constant2 : Constant  Value=15
  Data Type Conversion : DataTypeConversion  OutDataTypeStr=single  SaturateOnIntegerOverflow=off  RndMeth=Floor
  Data Type Conversion1 : DataTypeConversion  OutDataTypeStr=single  SaturateOnIntegerOverflow=off  RndMeth=Floor
  Data Type Conversion2 : DataTypeConversion  OutDataTypeStr=single  SaturateOnIntegerOverflow=off  RndMeth=Floor
  Demux1 : Demux  Outputs=8
  Gain : Gain  Gain=2*12.5/65535  RndMeth=Round
  Gain1 : Gain  Gain=2*45/4095  RndMeth=Round
  Gain2 : Gain  Gain=2*15/4095  RndMeth=Round
  Mux : Mux  Inputs=2
  Subsystem : Subsystem
  Sum : Sum  Inputs=|+-
  Sum1 : Sum  Inputs=|+-
  Sum2 : Sum  Inputs=|+-
  Terminator : Terminator
  Terminator3 : Terminator
  position : Outport
  speed : Outport  Port=2
  torque : Outport  Port=3
  wires:
  Demux1/1 -> Terminator3/1  "ID"
  Demux1/7 -> Mux/1
  Demux1/8 -> Mux/2
  Demux1/2 -> Subsystem/1(In1)
  Demux1/3 -> Subsystem/2(In2)
  Demux1/4 -> Subsystem/3(In3)
  Demux1/5 -> Subsystem/4(In4)
  Demux1/6 -> Subsystem/5(In5)
  Subsystem/1(Out1) -> Data Type Conversion/1
  Gain/1 -> Sum/1
  Constant/1 -> Sum/2
  Data Type Conversion/1 -> Gain/1
  Gain1/1 -> Sum1/1
  Data Type Conversion1/1 -> Gain1/1
  Constant1/1 -> Sum1/2
  Gain2/1 -> Sum2/1
  Data Type Conversion2/1 -> Gain2/1
  Constant2/1 -> Sum2/2
  Subsystem/2(Out2) -> Data Type Conversion1/1
  Subsystem/3(Out3) -> Data Type Conversion2/1
  Sum2/1 -> torque/1  "torque"
  Mux/1 -> Terminator/1
  Data/1 -> Demux1/1
  Sum/1 -> position/1  "position"
  Sum1/1 -> speed/1  "speed"

== system hip_controller_2026_03_03/Subsystem6/Left Motor Velocity/Subsystem/CAN Pack1 ==
  Position : Inport
  Velocity : Inport  Port=2
  Kp : Inport  Port=3
  Kd : Inport  Port=4
  Torque : Inport  Port=5
  Constant3 : Constant  Value=-12.5  OutDataTypeStr=single
  Constant4 : Constant  Value=-45  OutDataTypeStr=single
  Constant5 : Constant  Value=-15  OutDataTypeStr=single
  Gain : Gain  Gain=65535/(2*12.5)  OutDataTypeStr=uint16  RndMeth=Round
  Gain3 : Gain  Gain=4095/(2*45)  OutDataTypeStr=fixdt(0,12,0)  RndMeth=Round
  Gain4 : Gain  Gain=4095/500  OutDataTypeStr=fixdt(0,12,0)  RndMeth=Round
  Gain5 : Gain  Gain=4095/5  OutDataTypeStr=fixdt(0,12,0)  RndMeth=Round
  Gain6 : Gain  Gain=4095/(2*15)  OutDataTypeStr=fixdt(0,12,0)  RndMeth=Round
  Subsystem : Subsystem
  Sum3 : Sum  Inputs=|+-
  Sum4 : Sum  Inputs=|+-
  Sum5 : Sum  Inputs=|+-
  Vector Concatenate : Concatenate  NumInputs=8
  CAN Data : Outport
  wires:
  Velocity/1 -> Sum4/1
  Kp/1 -> Gain4/1
  Kd/1 -> Gain5/1
  Vector Concatenate/1 -> CAN Data/1
  Constant3/1 -> Sum3/2
  Sum3/1 -> Gain/1  "position"
  Position/1 -> Sum3/1
  Constant4/1 -> Sum4/2
  Constant5/1 -> Sum5/2
  Sum5/1 -> Gain6/1  "torque"
  Torque/1 -> Sum5/1
  Sum4/1 -> Gain3/1  "speed"
  Gain/1 -> Subsystem/1(p_int)
  Gain3/1 -> Subsystem/2(v_int)
  Gain4/1 -> Subsystem/3(kp_int)
  Gain5/1 -> Subsystem/4(kd_int)
  Gain6/1 -> Subsystem/5(t_int)
  Subsystem/1(Out2) -> Vector Concatenate/1
  Subsystem/2(Out1) -> Vector Concatenate/2
  Subsystem/4(Out4) -> Vector Concatenate/4
  Subsystem/5(Out5) -> Vector Concatenate/5
  Subsystem/6(Out6) -> Vector Concatenate/6
  Subsystem/7(Out7) -> Vector Concatenate/7
  Subsystem/3(Out3) -> Vector Concatenate/3
  Subsystem/8(Out8) -> Vector Concatenate/8

== system hip_controller_2026_03_03/Subsystem6/Left Motor Velocity/Subsystem/Subsystem2 ==
  Enable : Inport
  Velocity : Inport  Port=2
  Mux1 : Mux  Inputs=5
  Subsystem : Subsystem
  Subsystem2 : Subsystem
  Enter_motor_mode : Outport
  Velocity_value : Outport  Port=2
  wires:
  Subsystem2/3(Out3) -> Mux1/3
  Subsystem2/2(Out2) -> Mux1/2
  Subsystem2/4(Out4) -> Mux1/4
  Subsystem2/1(Out1) -> Mux1/1
  Subsystem/1(Out1) -> Velocity_value/1
  Mux1/1 -> Enter_motor_mode/1
  Enable/1 -> Mux1/5
  Velocity/1 -> Subsystem/1(In1)

== system hip_controller_2026_03_03/Subsystem6/Right Motor Velocity/Motor Actual Position Receive/CHINESE CORRECTION ==
  position : Inport
  Enable : EnablePort  StatesWhenEnabling=reset
  Abs : Abs  SaturateOnIntegerOverflow=off
  Constant2 : Constant
  Constant3 : Constant  Value=0
  Memory : Memory
  Subsystem : Subsystem
  Sum : Sum  Inputs=|+-
  Sum1 : Sum  Inputs=+-
  Switch1 : Switch  Criteria=u2 > Threshold  Threshold=20  SaturateOnIntegerOverflow=off  InputSameDT=off
  Out1 : Outport
  wires:
  Constant2/1 -> Switch1/1
  position/1 -> Sum1/1, Sum/1, Memory/1
  Sum/1 -> Abs/1, Subsystem/1(In1)
  Sum1/1 -> Out1/1
  Abs/1 -> Switch1/2
  Constant3/1 -> Switch1/3
  Switch1/1 -> Subsystem/Enable
  Memory/1 -> Sum/2
  Subsystem/1(Out1) -> Sum1/2

== system hip_controller_2026_03_03/Subsystem6/Right Motor Velocity/Motor Actual Position Receive/Unpack2 ==
  Data : Inport
  Constant : Constant  Value=12.5
  Constant1 : Constant  Value=45
  Constant2 : Constant  Value=15
  Data Type Conversion : DataTypeConversion  OutDataTypeStr=single  SaturateOnIntegerOverflow=off  RndMeth=Floor
  Data Type Conversion1 : DataTypeConversion  OutDataTypeStr=single  SaturateOnIntegerOverflow=off  RndMeth=Floor
  Data Type Conversion2 : DataTypeConversion  OutDataTypeStr=single  SaturateOnIntegerOverflow=off  RndMeth=Floor
  Demux1 : Demux  Outputs=8
  Gain : Gain  Gain=2*12.5/65535  RndMeth=Round
  Gain1 : Gain  Gain=2*45/4095  RndMeth=Round
  Gain2 : Gain  Gain=2*15/4095  RndMeth=Round
  Mux : Mux  Inputs=2
  Subsystem : Subsystem
  Sum : Sum  Inputs=|+-
  Sum1 : Sum  Inputs=|+-
  Sum2 : Sum  Inputs=|+-
  Terminator : Terminator
  Terminator3 : Terminator
  position : Outport
  speed : Outport  Port=2
  torque : Outport  Port=3
  wires:
  Demux1/1 -> Terminator3/1  "ID"
  Demux1/7 -> Mux/1
  Demux1/8 -> Mux/2
  Demux1/2 -> Subsystem/1(In1)
  Demux1/3 -> Subsystem/2(In2)
  Demux1/4 -> Subsystem/3(In3)
  Demux1/5 -> Subsystem/4(In4)
  Demux1/6 -> Subsystem/5(In5)
  Subsystem/1(Out1) -> Data Type Conversion/1
  Gain/1 -> Sum/1
  Constant/1 -> Sum/2
  Data Type Conversion/1 -> Gain/1
  Gain1/1 -> Sum1/1
  Data Type Conversion1/1 -> Gain1/1
  Constant1/1 -> Sum1/2
  Gain2/1 -> Sum2/1
  Data Type Conversion2/1 -> Gain2/1
  Constant2/1 -> Sum2/2
  Subsystem/2(Out2) -> Data Type Conversion1/1
  Subsystem/3(Out3) -> Data Type Conversion2/1
  Sum2/1 -> torque/1  "torque"
  Mux/1 -> Terminator/1
  Data/1 -> Demux1/1
  Sum/1 -> position/1  "position"
  Sum1/1 -> speed/1  "speed"
